simulink model "Copy_of_sm_car_test_ggv_new"  (R2026a)
settings: Solver=ode23t  StopTime=300  MaxStep=0.4  AbsTol=1e-3  EnableMultiTasking=on
PreLoadFcn:
  | % PreLoadFcn Removed for GGV Sweep
PostLoadFcn:
  | % PostLoadFcn Removed for GGV Sweep
InitFcn:
  | sm_car_config_camera;
  | Vehicle = sm_car_vehcfg_checkConfig(Vehicle);
  | sm_car_check_tire_model(bdroot);
StartFcn:
  | tic;
StopFcn:
  | Elapsed_Sim_Time = toc;
  | % disp(['Elapsed Sim Time = ' num2str(Elapsed_Sim_Time)]);
undefined symbols (not defined in the file): acc_theta, accel_ramp_rate, Axle1D, AxleIn, Camera, Control, drag_frc, Driver, Init, lift_frc, Maneuver, Pedal, Scene, ShaftL1, ShaftL2, ShaftR1, ShaftR2, Visual, X, xy_data_car_side, Y, Z
libraries: sm_lib x272, fl_lib x171, nesl_utility x139, simulink x58, simulink_extras x14, sdl_lib x14, SimscapeFluids_lib x7, dspsigops x4, Damper_Element x4, Tire_1x2x x4, ee_lib x3, Scene_Utilities x3
(part 10 of 21)

== system Copy_of_sm_car_test_ggv_new/World/Scene/CRG Hockenheim/Finish Line ==
  L1 : Subsystem  mask{square_lwh=[0.01 1 1]}
      mask prompts: square_lwh "Size [l w h] (m)"
  L2 : Subsystem  mask{square_lwh=[0.01 1 1]}
      mask prompts: square_lwh "Size [l w h] (m)"
  L3 : Subsystem  mask{square_lwh=[0.01 1 1]}
      mask prompts: square_lwh "Size [l w h] (m)"
  L4 : Subsystem  mask{square_lwh=[0.01 1 1]}
      mask prompts: square_lwh "Size [l w h] (m)"
  L5 : Subsystem  mask{square_lwh=[0.01 1 1]}
      mask prompts: square_lwh "Size [l w h] (m)"
  Post L : sm_lib/Body Elements/Cylindrical Solid  CylinderRadius=post_r  CylinderRadiusUnits=m  CylinderLength=post_h  CylinderLengthUnits=m  ExportEntireGeometry=off  InertiaType=CalculateFromGeometry  BasedOnType=Density  Density=1000  DensityUnits=kg/m^3  Mass=1  MassUnits=kg  CenterOfMass=[0 0 0]  CenterOfMassUnits=m  MomentsOfInertia=[1 1 1]  MomentsOfInertiaUnits=kg*m^2  ProductsOfInertia=[0 0 0]  ProductsOfInertiaUnits=kg*m^2  GraphicType=FromGeometry  MarkerShape=Sphere  MarkerSize=10  GraphicVisPropType=SimpleVisualProperties  GraphicDiffuseColor=post_clr  GraphicOpacity=post_opc  GraphicSpecularColor=[0.5 0.5 0.5 1.0]  GraphicAmbientColor=[0.15 0.15 0.15 1.0]  GraphicEmissiveColor=[0.0 0.0 0.0 1.0]  GraphicShininess=75  DoExposeReferenceFrame=off  SerializedFrames=<Frames><Frame><Id>Frame1</Id><Value><Name>B</Name><Origin><Source>GeometricFeature</Source><FeatureName>bottom surface</FeatureName></Origin><PrimaryAxis><DefinedDirection>+Z</DefinedDirection><Source>ReferenceFrame</Source><SourceDirection>+Z</SourceDirection><FeatureName></FeatureName></PrimaryAxis><SecondaryAxis><DefinedDirection>+X</DefinedDirection><Source>ReferenceFrame</Source><SourceDirection>+X</SourceDirection><FeatureName></FeatureName></SecondaryAxis></Value></Frame><Frame><Id>Frame2</Id><Value><Name>T</Name><Origin><Source>GeometricFeature</Source><FeatureName>top surface</FeatureName></Origin><PrimaryAxis><DefinedDirection>+Z</DefinedDirection><Source>ReferenceFrame</Source><SourceDirection>+Z</SourceDirection><FeatureName></FeatureName></PrimaryAxis><SecondaryAxis><DefinedDirection>+X</DefinedDirection><Source>ReferenceFrame</Source><SourceDirection>+X</SourceDirection><FeatureName></FeatureName></SecondaryAxis></Value></Frame></Frames>
  Post R : sm_lib/Body Elements/Cylindrical Solid  CylinderRadius=post_r  CylinderRadiusUnits=m  CylinderLength=post_h  CylinderLengthUnits=m  ExportEntireGeometry=off  InertiaType=CalculateFromGeometry  BasedOnType=Density  Density=1000  DensityUnits=kg/m^3  Mass=1  MassUnits=kg  CenterOfMass=[0 0 0]  CenterOfMassUnits=m  MomentsOfInertia=[1 1 1]  MomentsOfInertiaUnits=kg*m^2  ProductsOfInertia=[0 0 0]  ProductsOfInertiaUnits=kg*m^2  GraphicType=FromGeometry  MarkerShape=Sphere  MarkerSize=10  GraphicVisPropType=SimpleVisualProperties  GraphicDiffuseColor=post_clr  GraphicOpacity=post_opc  GraphicSpecularColor=[0.5 0.5 0.5 1.0]  GraphicAmbientColor=[0.15 0.15 0.15 1.0]  GraphicEmissiveColor=[0.0 0.0 0.0 1.0]  GraphicShininess=75  DoExposeReferenceFrame=off  SerializedFrames=<Frames><Frame><Id>Frame1</Id><Value><Name>B</Name><Origin><Source>GeometricFeature</Source><FeatureName>bottom surface</FeatureName></Origin><PrimaryAxis><DefinedDirection>+Z</DefinedDirection><Source>ReferenceFrame</Source><SourceDirection>+Z</SourceDirection><FeatureName></FeatureName></PrimaryAxis><SecondaryAxis><DefinedDirection>+X</DefinedDirection><Source>ReferenceFrame</Source><SourceDirection>+X</SourceDirection><FeatureName></FeatureName></SecondaryAxis></Value></Frame><Frame><Id>Frame2</Id><Value><Name>T</Name><Origin><Source>GeometricFeature</Source><FeatureName>top surface</FeatureName></Origin><PrimaryAxis><DefinedDirection>+Z</DefinedDirection><Source>ReferenceFrame</Source><SourceDirection>+Z</SourceDirection><FeatureName></FeatureName></PrimaryAxis><SecondaryAxis><DefinedDirection>+X</DefinedDirection><Source>ReferenceFrame</Source><SourceDirection>+X</SourceDirection><FeatureName></FeatureName></SecondaryAxis></Value></Frame></Frames>
  R1 : Subsystem  mask{square_lwh=[0.01 1 1]}
      mask prompts: square_lwh "Size [l w h] (m)"
  R2 : Subsystem  mask{square_lwh=[0.01 1 1]}
      mask prompts: square_lwh "Size [l w h] (m)"
  R3 : Subsystem  mask{square_lwh=[0.01 1 1]}
      mask prompts: square_lwh "Size [l w h] (m)"
  R4 : Subsystem  mask{square_lwh=[0.01 1 1]}
      mask prompts: square_lwh "Size [l w h] (m)"
  R5 : Subsystem  mask{square_lwh=[0.01 1 1]}
      mask prompts: square_lwh "Size [l w h] (m)"
  Transform Orient Line : sm_lib/Frames and Transforms/Rigid Transform  RotationMethod=RotationSequence  FollAlignAxisA=+X  BaseAlignAxisA=+Y  FollAlignAxisB=+Y  BaseAlignAxisB=+Z  RotationStandardAxis=+Z  RotationAngle=0  RotationAngleUnits=deg  RotationArbitraryAxis=[0 0 1]  RotationSequenceAxes=FollowerAxes  RotationSequence=ZYX  RotationSequenceAngles=[offset_yaw offset_pitch offset_roll]  RotationSequenceAnglesUnits=rad  RotationMatrix=[1 0 0; 0 1 0; 0 0 1]  Quaternion=[1 0 0 0]  TranslationMethod=Cartesian  TranslationCartesianOffset=offset_xyz  TranslationCartesianOffsetUnits=m  TranslationStandardAxis=+Z  TranslationStandardOffset=0  TranslationStandardOffsetUnits=m  TranslationROffset=0  TranslationROffsetUnits=m  TranslationThetaOffset=0  TranslationThetaOffsetUnits=deg  TranslationZOffset=0  TranslationZOffsetUnits=m
  Transform Post L : sm_lib/Frames and Transforms/Rigid Transform  RotationMethod=StandardAxis  FollAlignAxisA=+X  BaseAlignAxisA=+Y  FollAlignAxisB=+Y  BaseAlignAxisB=+Z  RotationStandardAxis=+Y  RotationAngle=0.0  RotationAngleUnits=deg  RotationArbitraryAxis=[0 0 1]  RotationSequenceAxes=FollowerAxes  RotationSequence=XYX  RotationSequenceAngles=[0 0 0]  RotationSequenceAnglesUnits=deg  RotationMatrix=[1 0 0; 0 1 0; 0 0 1]  Quaternion=[1 0 0 0]  TranslationMethod=StandardAxis  TranslationCartesianOffset=[0 0 0]  TranslationCartesianOffsetUnits=m  TranslationStandardAxis=+Y  TranslationStandardOffset=line_w/2  TranslationStandardOffsetUnits=m  TranslationROffset=0  TranslationROffsetUnits=m  TranslationThetaOffset=0  TranslationThetaOffsetUnits=deg  TranslationZOffset=0  TranslationZOffsetUnits=m
  Transform Post R : sm_lib/Frames and Transforms/Rigid Transform  RotationMethod=StandardAxis  FollAlignAxisA=+X  BaseAlignAxisA=+Y  FollAlignAxisB=+Y  BaseAlignAxisB=+Z  RotationStandardAxis=+Y  RotationAngle=0.0  RotationAngleUnits=deg  RotationArbitraryAxis=[0 0 1]  RotationSequenceAxes=FollowerAxes  RotationSequence=XYX  RotationSequenceAngles=[0 0 0]  RotationSequenceAnglesUnits=deg  RotationMatrix=[1 0 0; 0 1 0; 0 0 1]  Quaternion=[1 0 0 0]  TranslationMethod=StandardAxis  TranslationCartesianOffset=[0 0 0]  TranslationCartesianOffsetUnits=m  TranslationStandardAxis=+Y  TranslationStandardOffset=line_w/2  TranslationStandardOffsetUnits=m  TranslationROffset=0  TranslationROffsetUnits=m  TranslationThetaOffset=0  TranslationThetaOffsetUnits=deg  TranslationZOffset=0  TranslationZOffsetUnits=m
  W : PMIOPort  Side=Left
  connections:
  Post R/RConn1 -- R1/RConn1
  R2/RConn1 -- R1/LConn1
  L2/RConn1 -- L3/LConn1
  R4/RConn1 -- R3/LConn1
  Transform Post R/LConn1 -- Post R/LConn1
  L3/RConn1 -- L4/LConn1
  Post L/LConn1 -- Transform Post L/RConn1
  W/RConn1 -- Transform Orient Line/LConn1
  R2/LConn1 -- R3/RConn1
  L5/LConn1 -- L4/RConn1
  R5/RConn1 -- R4/LConn1
  L1/RConn1 -- L2/LConn1
  L1/LConn1 -- Post L/RConn1
  Transform Post L/LConn1 -- Transform Orient Line/RConn1 -- Transform Post R/RConn1

== system Copy_of_sm_car_test_ggv_new/World/Scene/CRG Hockenheim/STL Geometry Centerline ==
  Geometry : sm_lib/Body Elements/File Solid  ExtGeomFileName=CRG_Hockenheim_centerline.stl  UnitType=Custom  ExtGeomFileUnits=m  StepReaderType=HEX  ExportConvexHullGeometry=off  InertiaType=Custom  BasedOnType=DensityFromFile  Density=1000  DensityUnits=kg/m^3  Mass=1  MassUnits=kg  CenterOfMass=[0 0 0]  CenterOfMassUnits=m  MomentsOfInertia=[1 1 1]  MomentsOfInertiaUnits=kg*m^2  ProductsOfInertia=[0 0 0]  ProductsOfInertiaUnits=kg*m^2  GraphicType=FromGeometry  MarkerShape=Sphere  MarkerSize=10  GraphicVisPropType=SimpleVisualProperties  GraphicDiffuseColor=stl_clr  GraphicOpacity=stl_opc  GraphicSpecularColor=[0.5 0.5 0.5 1.0]  GraphicAmbientColor=[0.15 0.15 0.15 1.0]  GraphicEmissiveColor=[0.0 0.0 0.0 1.0]  GraphicShininess=75  DoExposeReferenceFrame=on  SerializedFrames=<Frames/>
  Transform Geometry : sm_lib/Frames and Transforms/Rigid Transform  RotationMethod=RotationSequence  FollAlignAxisA=+X  BaseAlignAxisA=+Y  FollAlignAxisB=+Y  BaseAlignAxisB=+Z  RotationStandardAxis=+Z  RotationAngle=0  RotationAngleUnits=rad  RotationArbitraryAxis=[0 0 1]  RotationSequenceAxes=FollowerAxes  RotationSequence=ZYX  RotationSequenceAngles=[stl_yaw stl_pitch stl_roll]  RotationSequenceAnglesUnits=rad  RotationMatrix=[1 0 0; 0 1 0; 0 0 1]  Quaternion=[1 0 0 0]  TranslationMethod=Cartesian  TranslationCartesianOffset=[stl_x stl_y stl_z]  TranslationCartesianOffsetUnits=m  TranslationStandardAxis=+Z  TranslationStandardOffset=0  TranslationStandardOffsetUnits=m  TranslationROffset=0  TranslationROffsetUnits=m  TranslationThetaOffset=0  TranslationThetaOffsetUnits=deg  TranslationZOffset=0  TranslationZOffsetUnits=m
  W : PMIOPort  Side=Right
  connections:
  Geometry/RConn1 -- Transform Geometry/RConn1
  Transform Geometry/LConn1 -- W/RConn1

== system Copy_of_sm_car_test_ggv_new/World/Scene/CRG Hockenheim/STL Geometry Road ==
  Geometry : sm_lib/Body Elements/File Solid  ExtGeomFileName=CRG_Hockenheim.stl  UnitType=Custom  ExtGeomFileUnits=m  StepReaderType=HEX  ExportConvexHullGeometry=off  InertiaType=Custom  BasedOnType=DensityFromFile  Density=1000  DensityUnits=kg/m^3  Mass=1  MassUnits=kg  CenterOfMass=[0 0 0]  CenterOfMassUnits=m  MomentsOfInertia=[1 1 1]  MomentsOfInertiaUnits=kg*m^2  ProductsOfInertia=[0 0 0]  ProductsOfInertiaUnits=kg*m^2  GraphicType=FromGeometry  MarkerShape=Sphere  MarkerSize=10  GraphicVisPropType=SimpleVisualProperties  GraphicDiffuseColor=stl_clr  GraphicOpacity=stl_opc  GraphicSpecularColor=[0.5 0.5 0.5 1.0]  GraphicAmbientColor=[0.15 0.15 0.15 1.0]  GraphicEmissiveColor=[0.0 0.0 0.0 1.0]  GraphicShininess=75  DoExposeReferenceFrame=on  SerializedFrames=<Frames/>
  Transform Geometry : sm_lib/Frames and Transforms/Rigid Transform  RotationMethod=RotationSequence  FollAlignAxisA=+X  BaseAlignAxisA=+Y  FollAlignAxisB=+Y  BaseAlignAxisB=+Z  RotationStandardAxis=+Z  RotationAngle=0  RotationAngleUnits=rad  RotationArbitraryAxis=[0 0 1]  RotationSequenceAxes=FollowerAxes  RotationSequence=ZYX  RotationSequenceAngles=[stl_yaw stl_pitch stl_roll]  RotationSequenceAnglesUnits=rad  RotationMatrix=[1 0 0; 0 1 0; 0 0 1]  Quaternion=[1 0 0 0]  TranslationMethod=Cartesian  TranslationCartesianOffset=[stl_x stl_y stl_z]  TranslationCartesianOffsetUnits=m  TranslationStandardAxis=+Z  TranslationStandardOffset=0  TranslationStandardOffsetUnits=m  TranslationROffset=0  TranslationROffsetUnits=m  TranslationThetaOffset=0  TranslationThetaOffsetUnits=deg  TranslationZOffset=0  TranslationZOffsetUnits=m
  W : PMIOPort  Side=Right
  connections:
  Geometry/RConn1 -- Transform Geometry/RConn1
  Transform Geometry/LConn1 -- W/RConn1

== system Copy_of_sm_car_test_ggv_new/World/Scene/CRG Hockenheim F/Finish Line ==
  L1 : Subsystem  mask{square_lwh=[0.01 1 1]}
      mask prompts: square_lwh "Size [l w h] (m)"
  L2 : Subsystem  mask{square_lwh=[0.01 1 1]}
      mask prompts: square_lwh "Size [l w h] (m)"
  L3 : Subsystem  mask{square_lwh=[0.01 1 1]}
      mask prompts: square_lwh "Size [l w h] (m)"
  L4 : Subsystem  mask{square_lwh=[0.01 1 1]}
      mask prompts: square_lwh "Size [l w h] (m)"
  L5 : Subsystem  mask{square_lwh=[0.01 1 1]}
      mask prompts: square_lwh "Size [l w h] (m)"
  Post L : sm_lib/Body Elements/Cylindrical Solid  CylinderRadius=post_r  CylinderRadiusUnits=m  CylinderLength=post_h  CylinderLengthUnits=m  ExportEntireGeometry=off  InertiaType=CalculateFromGeometry  BasedOnType=Density  Density=1000  DensityUnits=kg/m^3  Mass=1  MassUnits=kg  CenterOfMass=[0 0 0]  CenterOfMassUnits=m  MomentsOfInertia=[1 1 1]  MomentsOfInertiaUnits=kg*m^2  ProductsOfInertia=[0 0 0]  ProductsOfInertiaUnits=kg*m^2  GraphicType=FromGeometry  MarkerShape=Sphere  MarkerSize=10  GraphicVisPropType=SimpleVisualProperties  GraphicDiffuseColor=post_clr  GraphicOpacity=post_opc  GraphicSpecularColor=[0.5 0.5 0.5 1.0]  GraphicAmbientColor=[0.15 0.15 0.15 1.0]  GraphicEmissiveColor=[0.0 0.0 0.0 1.0]  GraphicShininess=75  DoExposeReferenceFrame=off  SerializedFrames=<Frames><Frame><Id>Frame1</Id><Value><Name>B</Name><Origin><Source>GeometricFeature</Source><FeatureName>bottom surface</FeatureName></Origin><PrimaryAxis><DefinedDirection>+Z</DefinedDirection><Source>ReferenceFrame</Source><SourceDirection>+Z</SourceDirection><FeatureName></FeatureName></PrimaryAxis><SecondaryAxis><DefinedDirection>+X</DefinedDirection><Source>ReferenceFrame</Source><SourceDirection>+X</SourceDirection><FeatureName></FeatureName></SecondaryAxis></Value></Frame><Frame><Id>Frame2</Id><Value><Name>T</Name><Origin><Source>GeometricFeature</Source><FeatureName>top surface</FeatureName></Origin><PrimaryAxis><DefinedDirection>+Z</DefinedDirection><Source>ReferenceFrame</Source><SourceDirection>+Z</SourceDirection><FeatureName></FeatureName></PrimaryAxis><SecondaryAxis><DefinedDirection>+X</DefinedDirection><Source>ReferenceFrame</Source><SourceDirection>+X</SourceDirection><FeatureName></FeatureName></SecondaryAxis></Value></Frame></Frames>
  Post R : sm_lib/Body Elements/Cylindrical Solid  CylinderRadius=post_r  CylinderRadiusUnits=m  CylinderLength=post_h  CylinderLengthUnits=m  ExportEntireGeometry=off  InertiaType=CalculateFromGeometry  BasedOnType=Density  Density=1000  DensityUnits=kg/m^3  Mass=1  MassUnits=kg  CenterOfMass=[0 0 0]  CenterOfMassUnits=m  MomentsOfInertia=[1 1 1]  MomentsOfInertiaUnits=kg*m^2  ProductsOfInertia=[0 0 0]  ProductsOfInertiaUnits=kg*m^2  GraphicType=FromGeometry  MarkerShape=Sphere  MarkerSize=10  GraphicVisPropType=SimpleVisualProperties  GraphicDiffuseColor=post_clr  GraphicOpacity=post_opc  GraphicSpecularColor=[0.5 0.5 0.5 1.0]  GraphicAmbientColor=[0.15 0.15 0.15 1.0]  GraphicEmissiveColor=[0.0 0.0 0.0 1.0]  GraphicShininess=75  DoExposeReferenceFrame=off  SerializedFrames=<Frames><Frame><Id>Frame1</Id><Value><Name>B</Name><Origin><Source>GeometricFeature</Source><FeatureName>bottom surface</FeatureName></Origin><PrimaryAxis><DefinedDirection>+Z</DefinedDirection><Source>ReferenceFrame</Source><SourceDirection>+Z</SourceDirection><FeatureName></FeatureName></PrimaryAxis><SecondaryAxis><DefinedDirection>+X</DefinedDirection><Source>ReferenceFrame</Source><SourceDirection>+X</SourceDirection><FeatureName></FeatureName></SecondaryAxis></Value></Frame><Frame><Id>Frame2</Id><Value><Name>T</Name><Origin><Source>GeometricFeature</Source><FeatureName>top surface</FeatureName></Origin><PrimaryAxis><DefinedDirection>+Z</DefinedDirection><Source>ReferenceFrame</Source><SourceDirection>+Z</SourceDirection><FeatureName></FeatureName></PrimaryAxis><SecondaryAxis><DefinedDirection>+X</DefinedDirection><Source>ReferenceFrame</Source><SourceDirection>+X</SourceDirection><FeatureName></FeatureName></SecondaryAxis></Value></Frame></Frames>
  R1 : Subsystem  mask{square_lwh=[0.01 1 1]}
      mask prompts: square_lwh "Size [l w h] (m)"
  R2 : Subsystem  mask{square_lwh=[0.01 1 1]}
      mask prompts: square_lwh "Size [l w h] (m)"
  R3 : Subsystem  mask{square_lwh=[0.01 1 1]}
      mask prompts: square_lwh "Size [l w h] (m)"
  R4 : Subsystem  mask{square_lwh=[0.01 1 1]}
      mask prompts: square_lwh "Size [l w h] (m)"
  R5 : Subsystem  mask{square_lwh=[0.01 1 1]}
      mask prompts: square_lwh "Size [l w h] (m)"
  Transform Orient Line : sm_lib/Frames and Transforms/Rigid Transform  RotationMethod=RotationSequence  FollAlignAxisA=+X  BaseAlignAxisA=+Y  FollAlignAxisB=+Y  BaseAlignAxisB=+Z  RotationStandardAxis=+Z  RotationAngle=0  RotationAngleUnits=deg  RotationArbitraryAxis=[0 0 1]  RotationSequenceAxes=FollowerAxes  RotationSequence=ZYX  RotationSequenceAngles=[offset_yaw offset_pitch offset_roll]  RotationSequenceAnglesUnits=rad  RotationMatrix=[1 0 0; 0 1 0; 0 0 1]  Quaternion=[1 0 0 0]  TranslationMethod=Cartesian  TranslationCartesianOffset=offset_xyz  TranslationCartesianOffsetUnits=m  TranslationStandardAxis=+Z  TranslationStandardOffset=0  TranslationStandardOffsetUnits=m  TranslationROffset=0  TranslationROffsetUnits=m  TranslationThetaOffset=0  TranslationThetaOffsetUnits=deg  TranslationZOffset=0  TranslationZOffsetUnits=m
  Transform Post L : sm_lib/Frames and Transforms/Rigid Transform  RotationMethod=StandardAxis  FollAlignAxisA=+X  BaseAlignAxisA=+Y  FollAlignAxisB=+Y  BaseAlignAxisB=+Z  RotationStandardAxis=+Y  RotationAngle=0.0  RotationAngleUnits=deg  RotationArbitraryAxis=[0 0 1]  RotationSequenceAxes=FollowerAxes  RotationSequence=XYX  RotationSequenceAngles=[0 0 0]  RotationSequenceAnglesUnits=deg  RotationMatrix=[1 0 0; 0 1 0; 0 0 1]  Quaternion=[1 0 0 0]  TranslationMethod=StandardAxis  TranslationCartesianOffset=[0 0 0]  TranslationCartesianOffsetUnits=m  TranslationStandardAxis=+Y  TranslationStandardOffset=line_w/2  TranslationStandardOffsetUnits=m  TranslationROffset=0  TranslationROffsetUnits=m  TranslationThetaOffset=0  TranslationThetaOffsetUnits=deg  TranslationZOffset=0  TranslationZOffsetUnits=m
  Transform Post R : sm_lib/Frames and Transforms/Rigid Transform  RotationMethod=StandardAxis  FollAlignAxisA=+X  BaseAlignAxisA=+Y  FollAlignAxisB=+Y  BaseAlignAxisB=+Z  RotationStandardAxis=+Y  RotationAngle=0.0  RotationAngleUnits=deg  RotationArbitraryAxis=[0 0 1]  RotationSequenceAxes=FollowerAxes  RotationSequence=XYX  RotationSequenceAngles=[0 0 0]  RotationSequenceAnglesUnits=deg  RotationMatrix=[1 0 0; 0 1 0; 0 0 1]  Quaternion=[1 0 0 0]  TranslationMethod=StandardAxis  TranslationCartesianOffset=[0 0 0]  TranslationCartesianOffsetUnits=m  TranslationStandardAxis=+Y  TranslationStandardOffset=line_w/2  TranslationStandardOffsetUnits=m  TranslationROffset=0  TranslationROffsetUnits=m  TranslationThetaOffset=0  TranslationThetaOffsetUnits=deg  TranslationZOffset=0  TranslationZOffsetUnits=m
  W : PMIOPort  Side=Left
  connections:
  Post R/RConn1 -- R1/RConn1
  R2/RConn1 -- R1/LConn1
  L2/RConn1 -- L3/LConn1
  R4/RConn1 -- R3/LConn1
  Transform Post R/LConn1 -- Post R/LConn1
  L3/RConn1 -- L4/LConn1
  Post L/LConn1 -- Transform Post L/RConn1
  W/RConn1 -- Transform Orient Line/LConn1
  R2/LConn1 -- R3/RConn1
  L5/LConn1 -- L4/RConn1
  R5/RConn1 -- R4/LConn1
  L1/RConn1 -- L2/LConn1
  L1/LConn1 -- Post L/RConn1
  Transform Post L/LConn1 -- Transform Orient Line/RConn1 -- Transform Post R/RConn1

== system Copy_of_sm_car_test_ggv_new/World/Scene/CRG Hockenheim F/STL Geometry Centerline ==
  Geometry : sm_lib/Body Elements/File Solid  ExtGeomFileName=CRG_Hockenheim_f_centerline.stl  UnitType=Custom  ExtGeomFileUnits=m  StepReaderType=HEX  ExportConvexHullGeometry=off  InertiaType=Custom  BasedOnType=DensityFromFile  Density=1000  DensityUnits=kg/m^3  Mass=1  MassUnits=kg  CenterOfMass=[0 0 0]  CenterOfMassUnits=m  MomentsOfInertia=[1 1 1]  MomentsOfInertiaUnits=kg*m^2  ProductsOfInertia=[0 0 0]  ProductsOfInertiaUnits=kg*m^2  GraphicType=FromGeometry  MarkerShape=Sphere  MarkerSize=10  GraphicVisPropType=SimpleVisualProperties  GraphicDiffuseColor=stl_clr  GraphicOpacity=stl_opc  GraphicSpecularColor=[0.5 0.5 0.5 1.0]  GraphicAmbientColor=[0.15 0.15 0.15 1.0]  GraphicEmissiveColor=[0.0 0.0 0.0 1.0]  GraphicShininess=75  DoExposeReferenceFrame=on  SerializedFrames=<Frames/>
  Transform Geometry : sm_lib/Frames and Transforms/Rigid Transform  RotationMethod=RotationSequence  FollAlignAxisA=+X  BaseAlignAxisA=+Y  FollAlignAxisB=+Y  BaseAlignAxisB=+Z  RotationStandardAxis=+Z  RotationAngle=0  RotationAngleUnits=rad  RotationArbitraryAxis=[0 0 1]  RotationSequenceAxes=FollowerAxes  RotationSequence=ZYX  RotationSequenceAngles=[stl_yaw stl_pitch stl_roll]  RotationSequenceAnglesUnits=rad  RotationMatrix=[1 0 0; 0 1 0; 0 0 1]  Quaternion=[1 0 0 0]  TranslationMethod=Cartesian  TranslationCartesianOffset=[stl_x stl_y stl_z]  TranslationCartesianOffsetUnits=m  TranslationStandardAxis=+Z  TranslationStandardOffset=0  TranslationStandardOffsetUnits=m  TranslationROffset=0  TranslationROffsetUnits=m  TranslationThetaOffset=0  TranslationThetaOffsetUnits=deg  TranslationZOffset=0  TranslationZOffsetUnits=m
  W : PMIOPort  Side=Right
  connections:
  Geometry/RConn1 -- Transform Geometry/RConn1
  Transform Geometry/LConn1 -- W/RConn1

== system Copy_of_sm_car_test_ggv_new/World/Scene/CRG Hockenheim F/STL Geometry Road ==
  Geometry : sm_lib/Body Elements/File Solid  ExtGeomFileName=CRG_Hockenheim_f.stl  UnitType=Custom  ExtGeomFileUnits=m  StepReaderType=HEX  ExportConvexHullGeometry=off  InertiaType=Custom  BasedOnType=DensityFromFile  Density=1000  DensityUnits=kg/m^3  Mass=1  MassUnits=kg  CenterOfMass=[0 0 0]  CenterOfMassUnits=m  MomentsOfInertia=[1 1 1]  MomentsOfInertiaUnits=kg*m^2  ProductsOfInertia=[0 0 0]  ProductsOfInertiaUnits=kg*m^2  GraphicType=FromGeometry  MarkerShape=Sphere  MarkerSize=10  GraphicVisPropType=SimpleVisualProperties  GraphicDiffuseColor=stl_clr  GraphicOpacity=stl_opc  GraphicSpecularColor=[0.5 0.5 0.5 1.0]  GraphicAmbientColor=[0.15 0.15 0.15 1.0]  GraphicEmissiveColor=[0.0 0.0 0.0 1.0]  GraphicShininess=75  DoExposeReferenceFrame=on  SerializedFrames=<Frames/>
  Transform Geometry : sm_lib/Frames and Transforms/Rigid Transform  RotationMethod=RotationSequence  FollAlignAxisA=+X  BaseAlignAxisA=+Y  FollAlignAxisB=+Y  BaseAlignAxisB=+Z  RotationStandardAxis=+Z  RotationAngle=0  RotationAngleUnits=rad  RotationArbitraryAxis=[0 0 1]  RotationSequenceAxes=FollowerAxes  RotationSequence=ZYX  RotationSequenceAngles=[stl_yaw stl_pitch stl_roll]  RotationSequenceAnglesUnits=rad  RotationMatrix=[1 0 0; 0 1 0; 0 0 1]  Quaternion=[1 0 0 0]  TranslationMethod=Cartesian  TranslationCartesianOffset=[stl_x stl_y stl_z]  TranslationCartesianOffsetUnits=m  TranslationStandardAxis=+Z  TranslationStandardOffset=0  TranslationStandardOffsetUnits=m  TranslationROffset=0  TranslationROffsetUnits=m  TranslationThetaOffset=0  TranslationThetaOffsetUnits=deg  TranslationZOffset=0  TranslationZOffsetUnits=m
  W : PMIOPort  Side=Right
  connections:
  Geometry/RConn1 -- Transform Geometry/RConn1
  Transform Geometry/LConn1 -- W/RConn1

== system Copy_of_sm_car_test_ggv_new/World/Scene/Plane Grid/Grid ==
  Mesh Lines x : Subsystem  mask(Rectangular Mesh){mesh_lenx=grid_x, mesh_leny=grid_y, mesh_hx=hole_wy, mesh_hy=hole_ly, mesh_numhx=1, mesh_numhy=grid_num_sq_y, mesh_thickness=grid_z, mesh_rho=7000, mesh_color=grid_clr, mesh_opc=grid_opc}
      mask prompts: mesh_thickness "Thickness (m)"; mesh_rho "Density (kg/m^3)"; mesh_color "Color [RGB]"; mesh_opc "Opacity (0-1)"
      mask help: Rectangular mesh. Define outer dimensions, dimensions of holes, and thickness. R port is at the CG. Thickness defines the distance of the F frame from the B frame along the z-axis.
      mask init:
      | mesh_xsec = Extr_Data_Mesh(mesh_lenx, mesh_leny, mesh_numhx, mesh_numhy, mesh_hx, mesh_hy);
      mask DialogControl Control12 Prompt: Plot Profile
      mask DialogControl Control12 Callback:
      | v = get_param(gcb,'MaskWSVariables');
      | getMaskValue = containers.Map({v.Name}',{v.Value}');
      | evalin('base',...
      |     sprintf('Extr_Data_Mesh(%s,%s,%s,%s,%s,%s,''%s'');',...
      |     num2str(getMaskValue('mesh_lenx')),...
      |     num2str(getMaskValue('mesh_leny')),...
      |     num2str(getMaskValue('mesh_numhx')),...
      |     num2str(getMaskValue('mesh_numhy')),...
      |     num2str(getMaskValue('mesh_hx')),...
      |     num2str(getMaskValue('mesh_hy')),'plot'));
      mask DialogControl Control7 Prompt: X
      mask DialogControl Control8 Prompt: Y
      mask DialogControl Control9 Prompt: Mesh Length (m)
      mask DialogControl Control11 Prompt: Hole Length (m)
      mask DialogControl Control10 Prompt: Number of Holes
      mask Display: image('Mesh_IMAGE.png');
  "Mesh Lines y " : Subsystem  mask(Rectangular Mesh){mesh_lenx=grid_x, mesh_leny=grid_y, mesh_hx=hole_lx, mesh_hy=hole_wx, mesh_numhx=grid_num_sq_x, mesh_numhy=1, mesh_thickness=grid_z, mesh_rho=7000, mesh_color=grid_clr, mesh_opc=grid_opc}
      mask prompts: mesh_thickness "Thickness (m)"; mesh_rho "Density (kg/m^3)"; mesh_color "Color [RGB]"; mesh_opc "Opacity (0-1)"
      mask help: Rectangular mesh. Define outer dimensions, dimensions of holes, and thickness. R port is at the CG. Thickness defines the distance of the F frame from the B frame along the z-axis.
      mask init:
      | mesh_xsec = Extr_Data_Mesh(mesh_lenx, mesh_leny, mesh_numhx, mesh_numhy, mesh_hx, mesh_hy);
      mask DialogControl Control12 Prompt: Plot Profile
      mask DialogControl Control12 Callback:
      | v = get_param(gcb,'MaskWSVariables');
      | getMaskValue = containers.Map({v.Name}',{v.Value}');
      | evalin('base',...
      |     sprintf('Extr_Data_Mesh(%s,%s,%s,%s,%s,%s,''%s'');',...
      |     num2str(getMaskValue('mesh_lenx')),...
      |     num2str(getMaskValue('mesh_leny')),...
      |     num2str(getMaskValue('mesh_numhx')),...
      |     num2str(getMaskValue('mesh_numhy')),...
      |     num2str(getMaskValue('mesh_hx')),...
      |     num2str(getMaskValue('mesh_hy')),'plot'));
      mask DialogControl Control7 Prompt: X
      mask DialogControl Control8 Prompt: Y
      mask DialogControl Control9 Prompt: Mesh Length (m)
      mask DialogControl Control11 Prompt: Hole Length (m)
      mask DialogControl Control10 Prompt: Number of Holes
      mask Display: image('Mesh_IMAGE.png');
  Reference Frame{,1..3} (4 alike) : sm_lib/Frames and Transforms/Reference Frame
  R : PMIOPort  Side=Left
  connections:
  Reference Frame3/RConn1 -- Mesh Lines x/RConn2
  "Mesh Lines y "/LConn1 -- Mesh Lines x/LConn1 -- R/RConn1
  "Mesh Lines y "/RConn1 -- Reference Frame/RConn1
  Reference Frame1/RConn1 -- "Mesh Lines y "/RConn2
  Reference Frame2/RConn1 -- Mesh Lines x/RConn1

== system Copy_of_sm_car_test_ggv_new/World/Scene/Plane Grid/Ground Plane ==
  Floor : sm_lib/Body Elements/Brick Solid  BrickDimensions=[gp_l, gp_w, gp_h]  BrickDimensionsUnits=m  ExportEntireGeometry=off  InertiaType=CalculateFromGeometry  BasedOnType=Density  Density=1000  DensityUnits=kg/m^3  Mass=1  MassUnits=kg  CenterOfMass=[0 0 0]  CenterOfMassUnits=m  MomentsOfInertia=[1 1 1]  MomentsOfInertiaUnits=kg*m^2  ProductsOfInertia=[0 0 0]  ProductsOfInertiaUnits=kg*m^2  GraphicType=FromGeometry  MarkerShape=Sphere  MarkerSize=10  GraphicVisPropType=SimpleVisualProperties  GraphicDiffuseColor=gp_clr  GraphicOpacity=gp_opc  GraphicSpecularColor=[0.5 0.5 0.5 1.0]  GraphicAmbientColor=[0.15 0.15 0.15 1.0]  GraphicEmissiveColor=[0.0 0.0 0.0 1.0]  GraphicShininess=75  DoExposeReferenceFrame=off  SerializedFrames=<Frames><Frame><Id>Frame1</Id><Value><Name>F</Name><Origin><Source>GeometricFeature</Source><FeatureName>+z surface</FeatureName></Origin><PrimaryAxis><DefinedDirection>+Z</DefinedDirection><Source>ReferenceFrame</Source><SourceDirection>+Z</SourceDirection><FeatureName></FeatureName></PrimaryAxis><SecondaryAxis><DefinedDirection>+X</DefinedDirection><Source>ReferenceFrame</Source><SourceDirection>+X</SourceDirection><FeatureName></FeatureName></SecondaryAxis></Value></Frame></Frames>
  W : PMIOPort  Side=Right
  connections:
  Floor/LConn1 -- W/RConn1

== system Copy_of_sm_car_test_ggv_new/World/Scene/Skidpad/Circle Inner L ==
  Solid : sm_lib/Body Elements/Extruded Solid  ExtrusionType=General  PolygonNumSides=3  PolygonOuterRadius=1  PolygonOuterRadiusUnits=m  ExportEntireGeometry=off  ExtrusionCrossSection=xy_data_circ  ExtrusionCrossSectionUnits=m  ExportConvexHullGeometry=off  ExtrusionLength=circ_h  ExtrusionLengthUnits=m  InertiaType=CalculateFromGeometry  BasedOnType=Density  Density=1000  DensityUnits=kg/m^3  Mass=1  MassUnits=kg  CenterOfMass=[0 0 0]  CenterOfMassUnits=m  MomentsOfInertia=[1 1 1]  MomentsOfInertiaUnits=kg*m^2  ProductsOfInertia=[1 1 1]  ProductsOfInertiaUnits=kg*m^2  GraphicType=FromGeometry  MarkerShape=Sphere  MarkerSize=10  GraphicVisPropType=SimpleVisualProperties  GraphicDiffuseColor=[1.0 1.0 0.8]  GraphicOpacity=1.0  GraphicSpecularColor=[0.5 0.5 0.5 1.0]  GraphicAmbientColor=[0.15 0.15 0.15 1.0]  GraphicEmissiveColor=[0.0 0.0 0.0 1.0]  GraphicShininess=75  DoExposeReferenceFrame=on  SerializedFrames=<Frames/>
  W : PMIOPort  Side=Right
  connections:
  Solid/RConn1 -- W/RConn1

== system Copy_of_sm_car_test_ggv_new/World/Scene/Skidpad/Circle Inner R ==
  Solid : sm_lib/Body Elements/Extruded Solid  ExtrusionType=General  PolygonNumSides=3  PolygonOuterRadius=1  PolygonOuterRadiusUnits=m  ExportEntireGeometry=off  ExtrusionCrossSection=xy_data_circ  ExtrusionCrossSectionUnits=m  ExportConvexHullGeometry=off  ExtrusionLength=circ_h  ExtrusionLengthUnits=m  InertiaType=CalculateFromGeometry  BasedOnType=Density  Density=1000  DensityUnits=kg/m^3  Mass=1  MassUnits=kg  CenterOfMass=[0 0 0]  CenterOfMassUnits=m  MomentsOfInertia=[1 1 1]  MomentsOfInertiaUnits=kg*m^2  ProductsOfInertia=[1 1 1]  ProductsOfInertiaUnits=kg*m^2  GraphicType=FromGeometry  MarkerShape=Sphere  MarkerSize=10  GraphicVisPropType=SimpleVisualProperties  GraphicDiffuseColor=[1.0 1.0 0.8]  GraphicOpacity=1.0  GraphicSpecularColor=[0.5 0.5 0.5 1.0]  GraphicAmbientColor=[0.15 0.15 0.15 1.0]  GraphicEmissiveColor=[0.0 0.0 0.0 1.0]  GraphicShininess=75  DoExposeReferenceFrame=on  SerializedFrames=<Frames/>
  W : PMIOPort  Side=Right
  connections:
  Solid/RConn1 -- W/RConn1

== system Copy_of_sm_car_test_ggv_new/World/Scene/Skidpad/Circle Outer L ==
  Solid : sm_lib/Body Elements/Extruded Solid  ExtrusionType=General  PolygonNumSides=3  PolygonOuterRadius=1  PolygonOuterRadiusUnits=m  ExportEntireGeometry=off  ExtrusionCrossSection=xy_data_circ  ExtrusionCrossSectionUnits=m  ExportConvexHullGeometry=off  ExtrusionLength=circ_h  ExtrusionLengthUnits=m  InertiaType=CalculateFromGeometry  BasedOnType=Density  Density=1000  DensityUnits=kg/m^3  Mass=1  MassUnits=kg  CenterOfMass=[0 0 0]  CenterOfMassUnits=m  MomentsOfInertia=[1 1 1]  MomentsOfInertiaUnits=kg*m^2  ProductsOfInertia=[1 1 1]  ProductsOfInertiaUnits=kg*m^2  GraphicType=FromGeometry  MarkerShape=Sphere  MarkerSize=10  GraphicVisPropType=SimpleVisualProperties  GraphicDiffuseColor=[1.0 1.0 0.8]  GraphicOpacity=1.0  GraphicSpecularColor=[0.5 0.5 0.5 1.0]  GraphicAmbientColor=[0.15 0.15 0.15 1.0]  GraphicEmissiveColor=[0.0 0.0 0.0 1.0]  GraphicShininess=75  DoExposeReferenceFrame=on  SerializedFrames=<Frames/>
  W : PMIOPort  Side=Right
  connections:
  Solid/RConn1 -- W/RConn1

== system Copy_of_sm_car_test_ggv_new/World/Scene/Skidpad/Circle Outer R ==
  Solid : sm_lib/Body Elements/Extruded Solid  ExtrusionType=General  PolygonNumSides=3  PolygonOuterRadius=1  PolygonOuterRadiusUnits=m  ExportEntireGeometry=off  ExtrusionCrossSection=xy_data_circ  ExtrusionCrossSectionUnits=m  ExportConvexHullGeometry=off  ExtrusionLength=circ_h  ExtrusionLengthUnits=m  InertiaType=CalculateFromGeometry  BasedOnType=Density  Density=1000  DensityUnits=kg/m^3  Mass=1  MassUnits=kg  CenterOfMass=[0 0 0]  CenterOfMassUnits=m  MomentsOfInertia=[1 1 1]  MomentsOfInertiaUnits=kg*m^2  ProductsOfInertia=[1 1 1]  ProductsOfInertiaUnits=kg*m^2  GraphicType=FromGeometry  MarkerShape=Sphere  MarkerSize=10  GraphicVisPropType=SimpleVisualProperties  GraphicDiffuseColor=[1.0 1.0 0.8]  GraphicOpacity=1.0  GraphicSpecularColor=[0.5 0.5 0.5 1.0]  GraphicAmbientColor=[0.15 0.15 0.15 1.0]  GraphicEmissiveColor=[0.0 0.0 0.0 1.0]  GraphicShininess=75  DoExposeReferenceFrame=on  SerializedFrames=<Frames/>
  W : PMIOPort  Side=Right
  connections:
  Solid/RConn1 -- W/RConn1

== system Copy_of_sm_car_test_ggv_new/World/Scene/Skidpad/Ground Plane ==
  Floor : sm_lib/Body Elements/Brick Solid  BrickDimensions=[gp_l, gp_w, gp_h]  BrickDimensionsUnits=m  ExportEntireGeometry=off  InertiaType=CalculateFromGeometry  BasedOnType=Density  Density=1000  DensityUnits=kg/m^3  Mass=1  MassUnits=kg  CenterOfMass=[0 0 0]  CenterOfMassUnits=m  MomentsOfInertia=[1 1 1]  MomentsOfInertiaUnits=kg*m^2  ProductsOfInertia=[0 0 0]  ProductsOfInertiaUnits=kg*m^2  GraphicType=FromGeometry  MarkerShape=Sphere  MarkerSize=10  GraphicVisPropType=SimpleVisualProperties  GraphicDiffuseColor=gp_clr  GraphicOpacity=gp_opc  GraphicSpecularColor=[0.5 0.5 0.5 1.0]  GraphicAmbientColor=[0.15 0.15 0.15 1.0]  GraphicEmissiveColor=[0.0 0.0 0.0 1.0]  GraphicShininess=75  DoExposeReferenceFrame=off  SerializedFrames=<Frames><Frame><Id>Frame1</Id><Value><Name>F</Name><Origin><Source>GeometricFeature</Source><FeatureName>+z surface</FeatureName></Origin><PrimaryAxis><DefinedDirection>+Z</DefinedDirection><Source>ReferenceFrame</Source><SourceDirection>+Z</SourceDirection><FeatureName></FeatureName></PrimaryAxis><SecondaryAxis><DefinedDirection>+X</DefinedDirection><Source>ReferenceFrame</Source><SourceDirection>+X</SourceDirection><FeatureName></FeatureName></SecondaryAxis></Value></Frame></Frames>
  W : PMIOPort  Side=Right
  connections:
  Floor/LConn1 -- W/RConn1

== system Copy_of_sm_car_test_ggv_new/Controller/Default/State Estimation/Sensor Noise Simulation/noise COG ==
  <vx> : Inport
  <COG> : Inport  Port=2
  Add1 : Sum
  Add2 : Sum
  Band-Limited White Noise1 : simulink/Sources/Band-Limited White Noise  Cov=[7e-3]  Ts=0.1  seed=[08854]
  Band-Limited White Noise2 : simulink/Sources/Band-Limited White Noise  Cov=[1.2e-5]  Ts=0.1  seed=[08854]
  Compare To Constant : simulink/Logic and Bit Operations/Compare To Constant  relop=<=  const=0.15  OutDataTypeStr=boolean
  Quantizer1 : Quantizer  QuantizationInterval=deg2rad(0.1)
  Quantizer2 : Quantizer  QuantizationInterval=deg2rad(0.1)
  Switch : Switch  Criteria=u2 ~= 0  SaturateOnIntegerOverflow=off  InputSameDT=off
  Zero-Order Hold1 : ZeroOrderHold  SampleTime=0.1
  Zero-Order Hold2 : ZeroOrderHold  SampleTime=0.1
  COG_n : Outport
  wires:
  Add2/1 -> Switch/3  "COG_n"
  <COG>/1 -> Quantizer1/1, Quantizer2/1
  Zero-Order Hold2/1 -> Add2/1
  Band-Limited White Noise2/1 -> Add2/2
  Quantizer2/1 -> Zero-Order Hold2/1
  <vx>/1 -> Compare To Constant/1
  Compare To Constant/1 -> Switch/2
  Quantizer1/1 -> Zero-Order Hold1/1
  Band-Limited White Noise1/1 -> Add1/2
  Zero-Order Hold1/1 -> Add1/1
  Add1/1 -> Switch/1  "COG_n"
  Switch/1 -> COG_n/1

== system Copy_of_sm_car_test_ggv_new/Controller/Default/State Estimation/Sensor Noise Simulation/noise a_x ==
  <w> : Inport
  Add2 : Sum
  Band-Limited White Noise2 : simulink/Sources/Band-Limited White Noise  Cov=[0.0024]  Ts=0.01  seed=[512361]
  Quantizer2 : Quantizer  QuantizationInterval=0.0047
  Zero-Order Hold2 : ZeroOrderHold  SampleTime=0.01
  a_x_n : Outport
  wires:
  Add2/1 -> a_x_n/1  "a_x_n"
  <w>/1 -> Quantizer2/1
  Zero-Order Hold2/1 -> Add2/1
  Band-Limited White Noise2/1 -> Add2/2
  Quantizer2/1 -> Zero-Order Hold2/1

== system Copy_of_sm_car_test_ggv_new/Controller/Default/State Estimation/Sensor Noise Simulation/noise a_y ==
  <w> : Inport
  Add2 : Sum
  Band-Limited White Noise2 : simulink/Sources/Band-Limited White Noise  Cov=[0.0024]  Ts=0.01  seed=[092756]
  Quantizer2 : Quantizer  QuantizationInterval=0.0047
  Zero-Order Hold2 : ZeroOrderHold  SampleTime=0.01
  a_y_n : Outport
  wires:
  Add2/1 -> a_y_n/1  "a_y_n"
  <w>/1 -> Quantizer2/1
  Zero-Order Hold2/1 -> Add2/1
  Band-Limited White Noise2/1 -> Add2/2
  Quantizer2/1 -> Zero-Order Hold2/1

== system Copy_of_sm_car_test_ggv_new/Controller/Default/State Estimation/Sensor Noise Simulation/noise omega_fl ==
  <w> : Inport
  Add2 : Sum
  Band-Limited White Noise2 : simulink/Sources/Band-Limited White Noise  Cov=[1e-4]  Ts=0.01  seed=[12451]
  Quantizer2 : Quantizer  QuantizationInterval=2 * pi / 25
  Zero-Order Hold2 : ZeroOrderHold  SampleTime=0.01
  omega_rl : Outport
  wires:
  Add2/1 -> omega_rl/1  "omega_rl"
  <w>/1 -> Quantizer2/1
  Zero-Order Hold2/1 -> Add2/1
  Band-Limited White Noise2/1 -> Add2/2
  Quantizer2/1 -> Zero-Order Hold2/1

== system Copy_of_sm_car_test_ggv_new/Controller/Default/State Estimation/Sensor Noise Simulation/noise omega_fr ==
  <w> : Inport
  Add3 : Sum
  Band-Limited White Noise3 : simulink/Sources/Band-Limited White Noise  Cov=[1e-4]  Ts=0.01  seed=[68595]
  Quantizer3 : Quantizer  QuantizationInterval=2 * pi / 25
  Zero-Order Hold3 : ZeroOrderHold  SampleTime=0.01
  omega_rr : Outport
  wires:
  Add3/1 -> omega_rr/1  "omega_rr"
  Band-Limited White Noise3/1 -> Add3/2
  Zero-Order Hold3/1 -> Add3/1
  <w>/1 -> Quantizer3/1
  Quantizer3/1 -> Zero-Order Hold3/1

== system Copy_of_sm_car_test_ggv_new/Controller/Default/State Estimation/Sensor Noise Simulation/noise omega_rl ==
  <w> : Inport
  Add : Sum
  Band-Limited White Noise : simulink/Sources/Band-Limited White Noise  Cov=[1e-4]  Ts=0.01  seed=[23341]
  Quantizer : Quantizer  QuantizationInterval=2 * pi / 94
  Zero-Order Hold : ZeroOrderHold  SampleTime=0.01
  omega_rl : Outport
  wires:
  Quantizer/1 -> Zero-Order Hold/1
  <w>/1 -> Quantizer/1
  Band-Limited White Noise/1 -> Add/2
  Add/1 -> omega_rl/1  "omega_rl"
  Zero-Order Hold/1 -> Add/1

== system Copy_of_sm_car_test_ggv_new/Controller/Default/State Estimation/Sensor Noise Simulation/noise omega_rr ==
  <w> : Inport
  Add1 : Sum
  Band-Limited White Noise1 : simulink/Sources/Band-Limited White Noise  Cov=[1e-4]  Ts=0.01  seed=[41245]
  Quantizer1 : Quantizer  QuantizationInterval=2 * pi / 94
  Zero-Order Hold1 : ZeroOrderHold  SampleTime=0.01
  omega_rr : Outport
  wires:
  Add1/1 -> omega_rr/1  "omega_rr"
  Quantizer1/1 -> Zero-Order Hold1/1
  <w>/1 -> Quantizer1/1
  Band-Limited White Noise1/1 -> Add1/2
  Zero-Order Hold1/1 -> Add1/1

== system Copy_of_sm_car_test_ggv_new/Controller/Default/State Estimation/Sensor Noise Simulation/noise v_gps ==
  <vz> : Inport
  <vx> : Inport  Port=2
  <vy> : Inport  Port=3
  Add : Sum  Inputs=+++
  Add2 : Sum
  Band-Limited White Noise2 : simulink/Sources/Band-Limited White Noise  Cov=[9e-4]  Ts=0.1  seed=[645743]
  Quantizer2 : Quantizer  QuantizationInterval=0.01
  Sqrt : Sqrt
  Square : Math  Operator=square
  Square1 : Math  Operator=square
  Square2 : Math  Operator=square
  Zero-Order Hold2 : ZeroOrderHold  SampleTime=0.1
  V_GPS_n : Outport
  wires:
  Quantizer2/1 -> Zero-Order Hold2/1
  Band-Limited White Noise2/1 -> Add2/2
  Zero-Order Hold2/1 -> Add2/1
  Sqrt/1 -> Quantizer2/1
  Add2/1 -> V_GPS_n/1  "V_GPS_n"
  <vz>/1 -> Square/1
  <vx>/1 -> Square1/1
  <vy>/1 -> Square2/1
  Add/1 -> Sqrt/1
  Square/1 -> Add/1
  Square1/1 -> Add/2
  Square2/1 -> Add/3

== system Copy_of_sm_car_test_ggv_new/Controller/Default/State Estimation/Sensor Noise Simulation/noise yaw ==
  <w> : Inport
  Add2 : Sum
  Band-Limited White Noise2 : simulink/Sources/Band-Limited White Noise  Cov=[1.2e-7]  Ts=0.01  seed=[211845]
  Quantizer2 : Quantizer  QuantizationInterval=deg2rad(0.1)
  Zero-Order Hold2 : ZeroOrderHold  SampleTime=0.01
  aYaw_n : Outport
  wires:
  Quantizer2/1 -> Zero-Order Hold2/1
  Band-Limited White Noise2/1 -> Add2/2
  Zero-Order Hold2/1 -> Add2/1
  <w>/1 -> Quantizer2/1
  Add2/1 -> aYaw_n/1  "aYaw_n"

== system Copy_of_sm_car_test_ggv_new/Controller/Default/State Estimation/Sensor Noise Simulation/noise yaw rate ==
  <w> : Inport
  Add2 : Sum
  Band-Limited White Noise2 : simulink/Sources/Band-Limited White Noise  Cov=[7.6e-7]  Ts=0.01  seed=[809953]
  Quantizer2 : Quantizer  QuantizationInterval=0.001
  Zero-Order Hold2 : ZeroOrderHold  SampleTime=0.01
  nYaw_n : Outport
  wires:
  Quantizer2/1 -> Zero-Order Hold2/1
  Band-Limited White Noise2/1 -> Add2/2
  Zero-Order Hold2/1 -> Add2/1
  <w>/1 -> Quantizer2/1
  Add2/1 -> nYaw_n/1  "nYaw_n"

== system Copy_of_sm_car_test_ggv_new/Controller/TrqVec 4Motor/Brake Control/ABS/Calculate Slip ==
  WhlSpd : Inport
  VehSpdEst : Inport  Port=2
  Abs : Abs  ZeroCross=off  SaturateOnIntegerOverflow=off
  Bus Creator : BusCreator  Inputs=4
  Bus Selector1 : BusSelector  OutputSignals=L1.v,R1.v,L2.v,R2.v
  Constant : Constant
  Demux : Demux
  Fcn{,1..3} (4 alike) : Fcn  Expr=abs(u(1)*u(2)-u(3))/u(3)
  Mux{,1..3} (4 alike) : Mux  Inputs=3
  Mux4 : Mux
  Mux5 : Mux
  Product : Product
  Saturation : Saturate  UpperLimit=inf  LowerLimit=eps  ZeroCross=off
  Saturation1 : Saturate  UpperLimit=1  LowerLimit=0
  Sign : Signum  ZeroCross=off
  Wheel Speeds and Slip : Scope  NumInputPorts=2
      settings: ActiveDisplayYMinimum=-11.64241  ActiveDisplayYMaximum=114.01232  DataLoggingVariableName=ScopeData2
  Slip : Outport  VectorParamsAs1DForOutWhenUnconnected=off
  wires:
  WhlSpd/1 -> Bus Selector1/1
  Bus Selector1/2 -> Mux4/2, Mux1/2  "<v>"
  Bus Selector1/4 -> Mux4/4, Mux3/2  "<v>"
  Bus Selector1/1 -> Mux4/1, Mux/2  "<v>"
  Bus Selector1/3 -> Mux4/3, Mux2/2  "<v>"
  Constant/1 -> Mux/1, Mux1/1, Mux3/1, Mux2/1
  VehSpdEst/1 -> Sign/1, Abs/1
  Demux/1 -> Bus Creator/1  "L1"
  Demux/2 -> Bus Creator/2  "R1"
  Demux/3 -> Bus Creator/3  "L2"
  Demux/4 -> Bus Creator/4  "R2"
  Bus Creator/1 -> Wheel Speeds and Slip/2, Slip/1  "Slip"
  Product/1 -> Mux3/3, Mux2/3, Mux1/3, Mux/3
  Abs/1 -> Saturation/1
  Saturation/1 -> Product/1
  Sign/1 -> Product/2
  Mux/1 -> Fcn/1
  Mux1/1 -> Fcn1/1
  Mux2/1 -> Fcn2/1
  Mux3/1 -> Fcn3/1
  Mux4/1 -> Wheel Speeds and Slip/1  "Wheel Speeds"
  Mux5/1 -> Saturation1/1
  Saturation1/1 -> Demux/1
  Fcn/1 -> Mux5/1  "L1"
  Fcn1/1 -> Mux5/2  "R1"
  Fcn2/1 -> Mux5/3  "L2"
  Fcn3/1 -> Mux5/4  "R2"

== system Copy_of_sm_car_test_ggv_new/Controller/TrqVec 4Motor/Brake Control/ABS/Sensor ==
  Body : Inport
  WhlSpd : Inport  Port=2
  Bus Creator{,3..5} (4 alike) : BusCreator  Inputs=1
  Bus Creator6 : BusCreator  Inputs=5
  Bus Selector : BusSelector  OutputSignals=vx,vy  OutputAsBus=on
  Bus Selector4 : BusSelector  OutputSignals=WhlL1.n,WhlR1.n,WhlL2.n,WhlR2.n,WhlL2.qxyz
  Gain : Gain  Gain=3.6*abs_tire_radiusF
  Gain1 : Gain  Gain=3.6*abs_tire_radiusF
  Gain2 : Gain  Gain=3.6*abs_tire_radiusR
  Gain3 : Gain  Gain=3.6*abs_tire_radiusR
  Gain4 : Gain  Gain=3.6
  Terminator1 : Terminator  Commented=on
  Vel in xy plane : Fcn  Expr=sqrt(u(1)^2+u(2)^2)
  missing tooth : Subsystem  Commented=on
  GroundSpd : Outport  VectorParamsAs1DForOutWhenUnconnected=off
  wires:
  Gain1/1 -> Bus Creator3/1  "v"
  missing tooth/1(Out1) -> Terminator1/1  "v"
  Gain2/1 -> Bus Creator4/1  "v"
  Bus Selector4/5 -> missing tooth/2(<qxyz>)  "<qxyz>"
  Bus Creator5/1 -> Bus Creator6/5  "R2"
  Gain3/1 -> Bus Creator5/1  "v"
  Bus Creator/1 -> Bus Creator6/2  "L1"
  Bus Selector4/2 -> Gain1/1  "<n>"
  Bus Creator4/1 -> Bus Creator6/4  "L2"
  Bus Selector4/3 -> Gain2/1, missing tooth/1(<omega>)  "<n>"
  Gain/1 -> Bus Creator/1  "v"
  Body/1 -> Bus Selector/1
  Bus Creator3/1 -> Bus Creator6/3  "R1"
  Gain4/1 -> Bus Creator6/1  "v"
  Bus Selector4/1 -> Gain/1  "<n>"
  Bus Selector4/4 -> Gain3/1  "<n>"
  WhlSpd/1 -> Bus Selector4/1
  Bus Creator6/1 -> GroundSpd/1
  Vel in xy plane/1 -> Gain4/1  "speed"
  Bus Selector/1 -> Vel in xy plane/1

== system Copy_of_sm_car_test_ggv_new/Controller/TrqVec 4Motor/Brake Control/ABS/Valve Control L1 ==
  Slip : Inport
  vSpdEst : Inport  Port=2
  Categorize Surface : Subsystem
  Code to Valves : Subsystem
  Demux : Demux  Outputs=2
  Logic : Stateflow chart  TreatAsAtomicUnit=on
  Mux : Mux  Inputs=2
  Product : Product
  Subsystem : Subsystem
  Subsystem1 : Subsystem
  Valve : Outport  VectorParamsAs1DForOutWhenUnconnected=off
  wires:
  Logic/1(Mod_State) -> Categorize Surface/1(Mod State), Code to Valves/1(C)
  Logic/2(Mod_Dur) -> Product/2
  Slip/1 -> Logic/1(Slip)
  Code to Valves/1(V) -> Product/1
  vSpdEst/1 -> Logic/2(vSpdEst)
  Product/1 -> Demux/1
  Demux/1 -> Subsystem/1(OnT)
  Demux/2 -> Subsystem1/1(OnT)
  Mux/1 -> Valve/1
  Subsystem/1(vSig) -> Mux/1, Categorize Surface/2(Apply Valve)
  Subsystem1/1(vSig) -> Mux/2

== system Copy_of_sm_car_test_ggv_new/Controller/TrqVec 4Motor/Brake Control/ABS/Valve Control L2 ==
  Slip : Inport
  vSpdEst : Inport  Port=2
  Categorize Surface : Subsystem
  Code to Valves : Subsystem
  Demux : Demux  Outputs=2
  Logic : Stateflow chart  TreatAsAtomicUnit=on
  Mux : Mux  Inputs=2
  Product : Product
  Subsystem : Subsystem
  Subsystem1 : Subsystem
  Valve : Outport  VectorParamsAs1DForOutWhenUnconnected=off
  wires:
  Logic/1(Mod_State) -> Categorize Surface/1(Mod State), Code to Valves/1(C)
  Logic/2(Mod_Dur) -> Product/2
  Slip/1 -> Logic/1(Slip)
  Code to Valves/1(V) -> Product/1
  vSpdEst/1 -> Logic/2(vSpdEst)
  Product/1 -> Demux/1
  Demux/1 -> Subsystem/1(OnT)
  Demux/2 -> Subsystem1/1(OnT)
  Mux/1 -> Valve/1
  Subsystem/1(vSig) -> Mux/1, Categorize Surface/2(Apply Valve)
  Subsystem1/1(vSig) -> Mux/2

== system Copy_of_sm_car_test_ggv_new/Controller/TrqVec 4Motor/Brake Control/ABS/Valve Control R1 ==
  Slip : Inport
  vSpdEst : Inport  Port=2
  Categorize Surface : Subsystem
  Code to Valves : Subsystem
  Demux : Demux  Outputs=2
  Logic : Stateflow chart  TreatAsAtomicUnit=on
  Mux : Mux  Inputs=2
  Product : Product
  Subsystem : Subsystem
  Subsystem1 : Subsystem
  Valve : Outport  VectorParamsAs1DForOutWhenUnconnected=off
  wires:
  Logic/1(Mod_State) -> Categorize Surface/1(Mod State), Code to Valves/1(C)
  Logic/2(Mod_Dur) -> Product/2
  Slip/1 -> Logic/1(Slip)
  Code to Valves/1(V) -> Product/1
  vSpdEst/1 -> Logic/2(vSpdEst)
  Product/1 -> Demux/1
  Demux/1 -> Subsystem/1(OnT)
  Demux/2 -> Subsystem1/1(OnT)
  Mux/1 -> Valve/1
  Subsystem/1(vSig) -> Mux/1, Categorize Surface/2(Apply Valve)
  Subsystem1/1(vSig) -> Mux/2

== system Copy_of_sm_car_test_ggv_new/Controller/TrqVec 4Motor/Brake Control/ABS/Valve Control R2 ==
  Slip : Inport
  vSpdEst : Inport  Port=2
  Categorize Surface : Subsystem
  Code to Valves : Subsystem
  Demux : Demux  Outputs=2
  Logic : Stateflow chart  TreatAsAtomicUnit=on
  Mux : Mux  Inputs=2
  Product : Product
  Subsystem : Subsystem
  Subsystem1 : Subsystem
  Valve : Outport  VectorParamsAs1DForOutWhenUnconnected=off
  wires:
  Logic/1(Mod_State) -> Categorize Surface/1(Mod State), Code to Valves/1(C)
  Logic/2(Mod_Dur) -> Product/2
  Slip/1 -> Logic/1(Slip)
  Code to Valves/1(V) -> Product/1
  vSpdEst/1 -> Logic/2(vSpdEst)
  Product/1 -> Demux/1
  Demux/1 -> Subsystem/1(OnT)
  Demux/2 -> Subsystem1/1(OnT)
  Mux/1 -> Valve/1
  Subsystem/1(vSig) -> Mux/1, Categorize Surface/2(Apply Valve)
  Subsystem1/1(vSig) -> Mux/2

== system Copy_of_sm_car_test_ggv_new/Controller/TrqVec 4Motor/Brake Control/ABS/Vehicle Speed ==
  Sensors : Inport
  Bus Selector : BusSelector  OutputSignals=v
  vSpdEst : Outport  VectorParamsAs1DForOutWhenUnconnected=off
  wires:
  Sensors/1 -> Bus Selector/1
  Bus Selector/1 -> vSpdEst/1  "<v>"

== system Copy_of_sm_car_test_ggv_new/Controller/TrqVec 4Motor/Power_TqVec/Torque Vectoring/Accel Torque Request ==
  note: Assumes both rear motors have same torque speed curve
  MotSpdL2 : Inport
  MotSpdR2 : Inport  Port=2
  MaxMotTrqVsSpdA1 : Lookup_n-D  NumberOfTableDimensions=1  BreakpointsForDimension1=Control.MotorL2.TorqueSpd.w.Value  Table=Control.MotorL2.TorqueSpd.trq.Value  ExtrapMethod=Clip  UseLastTableValue=on  InternalRulePriority=Speed  OutDataTypeStr=Inherit: Inherit from 'Table data'  RndMeth=Simplest
  Terminator : Terminator
  rads_to_rpm : Gain  Gain=30/pi
  rads_to_rpm1 : Gain  Gain=30/pi
  TrqMax : Outport  VectorParamsAs1DForOutWhenUnconnected=off
  wires:
  rads_to_rpm1/1 -> Terminator/1
  MotSpdR2/1 -> rads_to_rpm1/1
  MaxMotTrqVsSpdA1/1 -> TrqMax/1
  MotSpdL2/1 -> rads_to_rpm/1
  rads_to_rpm/1 -> MaxMotTrqVsSpdA1/1

== system Copy_of_sm_car_test_ggv_new/Controller/TrqVec 4Motor/Power_TqVec/Torque Vectoring/Enable ==
  note: Ramp up amount of torque vectoring over a range.
  note: Steer angle threshold to enable torque vectoring
  vx : Inport
  aSteerWheel : Inport  Port=2
  Abs : Abs  ZeroCross=off  SaturateOnIntegerOverflow=off
  Data Type Conversion : DataTypeConversion  OutDataTypeStr=double  SaturateOnIntegerOverflow=off  RndMeth=Floor
  Divide : Product  Inputs=*/
  Enable vx : simulink/Logic and Bit Operations/Compare To Constant  relop=>  const=vx_enable  OutDataTypeStr=boolean  ZeroCross=off
  Gain : Gain  Gain=0.25
  Product : Product
  Saturation : Saturate  UpperLimit=1  LowerLimit=0  ZeroCross=off
  Subtract : Sum  Inputs=+-
  const : Constant  Value=aSteerWheel_enable
  Enable : Outport  VectorParamsAs1DForOutWhenUnconnected=off
  wires:
  Gain/1 -> Divide/1
  Product/1 -> Enable/1
  Divide/1 -> Saturation/1
  Subtract/1 -> Gain/1
  Abs/1 -> Subtract/1
  Saturation/1 -> Product/2
  Data Type Conversion/1 -> Product/1
  Enable vx/1 -> Data Type Conversion/1
  const/1 -> Subtract/2, Divide/2
  aSteerWheel/1 -> Abs/1
  vx/1 -> Enable vx/1
